simulink model "seven"  (R2020b)
settings: Solver=VariableStepAuto  StartTime=0.0  StopTime=10.0  RelTol=1e-3
settings Model: Creator=Dell  LastModifiedBy=Dell

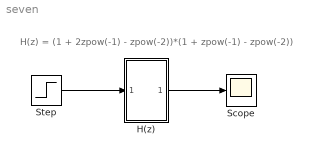
== system seven ==
  note: H(z) = (1 + 2zpow(-1) - zpow(-2))*(1 + zpow(-1) - zpow(-2))
  H(z) : Subsystem
  Scope : Scope
  Step : Step  SampleTime=0
  wires:
  Step/1 -> H(z)/1(In1)
  H(z)/1(Out1) -> Scope/1

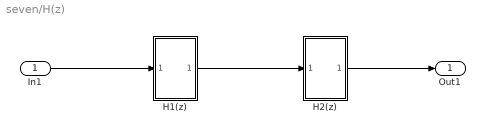
== system seven/H(z) ==
  In1 : Inport
  H1(z) : Subsystem
  H2(z) : Subsystem
  Out1 : Outport
  wires:
  H1(z)/1(Out1) -> H2(z)/1(In1)
  H2(z)/1(Out1) -> Out1/1
  In1/1 -> H1(z)/1(In1)

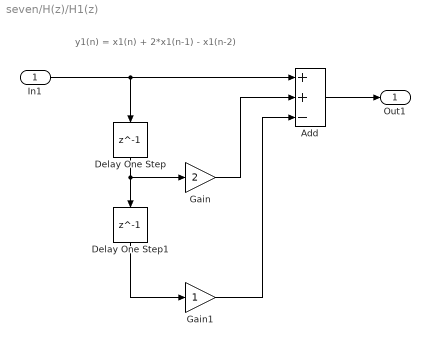
== system seven/H(z)/H1(z) ==
  note: y1(n) = x1(n) + 2*x1(n-1) - x1(n-2)
  In1 : Inport
  Add : Sum  Inputs=++-
  Delay One Step : Delay  DelayLength=1
  Delay One Step1 : Delay  DelayLength=1
  Gain : Gain  Gain=2
  Gain1 : Gain
  Out1 : Outport
  wires:
  Delay One Step1/1 -> Gain1/1
  In1/1 -> Delay One Step/1, Add/1
  Add/1 -> Out1/1
  Gain1/1 -> Add/3
  Gain/1 -> Add/2
  Delay One Step/1 -> Gain/1, Delay One Step1/1

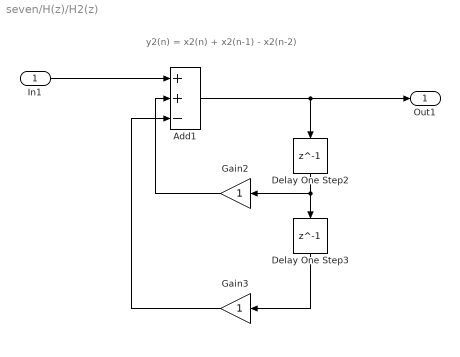
== system seven/H(z)/H2(z) ==
  note: y2(n) = x2(n) + x2(n-1) - x2(n-2)
  In1 : Inport
  Add1 : Sum  Inputs=++-
  Delay One Step2 : Delay  DelayLength=1
  Delay One Step3 : Delay  DelayLength=1
  Gain2 : Gain
  Gain3 : Gain
  Out1 : Outport
  wires:
  In1/1 -> Add1/1
  Add1/1 -> Out1/1, Delay One Step2/1
  Delay One Step2/1 -> Gain2/1, Delay One Step3/1
  Gain2/1 -> Add1/2
  Delay One Step3/1 -> Gain3/1
  Gain3/1 -> Add1/3
